simulink model "Filter"  (R2021a)
settings: Solver=VariableStepAuto  StartTime=0.0  StopTime=(len-1)*dt  FixedStep=0..005  RelTol=1e-3
values from neighbouring files (symbols this model uses):
  taos = 0.005    [Identify.m]    (also in Identify_time.m; Identify_wc.m)
  Wf = 10    [Identify.m]    (also in Identify_time.m; Identify_wc.m = Wf_list(i))
  zeta = 0.9    [Identify.m]    (also in Identify_time.m; Identify_wc.m)
settings Model: Creator=1  LastModifiedBy=1

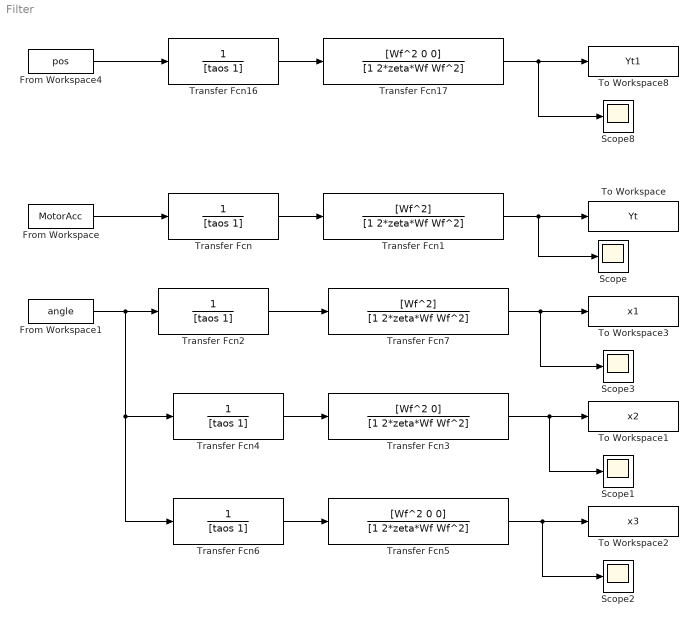
== system Filter ==
  From Workspace : FromWorkspace  VariableName=MotorAcc  OutDataTypeStr=double
  From Workspace1 : FromWorkspace  VariableName=angle  OutDataTypeStr=double
  From Workspace4 : FromWorkspace  VariableName=pos  OutDataTypeStr=double
  Scope{,1..3,8} (5 alike) : Scope
  To Workspace : ToWorkspace  VariableName=Yt  SampleTime=0.005
  To Workspace1 : ToWorkspace  VariableName=x2  SampleTime=0.005
  To Workspace2 : ToWorkspace  VariableName=x3  SampleTime=0.005
  To Workspace3 : ToWorkspace  VariableName=x1  SampleTime=0.005
  To Workspace8 : ToWorkspace  VariableName=Yt1  SampleTime=0.005
  Transfer Fcn{,2,4,6,16} (5 alike) : TransferFcn  Denominator=[taos 1]
  Transfer Fcn1 : TransferFcn  Numerator=[Wf^2]  Denominator=[1 2*zeta*Wf Wf^2]
  Transfer Fcn17 : TransferFcn  Numerator=[Wf^2 0 0]  Denominator=[1 2*zeta*Wf Wf^2]
  Transfer Fcn3 : TransferFcn  Numerator=[Wf^2 0]  Denominator=[1 2*zeta*Wf Wf^2]
  Transfer Fcn5 : TransferFcn  Numerator=[Wf^2 0 0]  Denominator=[1 2*zeta*Wf Wf^2]
  Transfer Fcn7 : TransferFcn  Numerator=[Wf^2]  Denominator=[1 2*zeta*Wf Wf^2]
  wires:
  From Workspace/1 -> Transfer Fcn/1
  Transfer Fcn7/1 -> Scope3/1, To Workspace3/1
  Transfer Fcn2/1 -> Transfer Fcn7/1
  From Workspace1/1 -> Transfer Fcn2/1, Transfer Fcn6/1, Transfer Fcn4/1
  Transfer Fcn/1 -> Transfer Fcn1/1
  Transfer Fcn1/1 -> Scope/1, To Workspace/1
  Transfer Fcn3/1 -> Scope1/1, To Workspace1/1
  Transfer Fcn4/1 -> Transfer Fcn3/1
  Transfer Fcn6/1 -> Transfer Fcn5/1
  Transfer Fcn5/1 -> Scope2/1, To Workspace2/1
  Transfer Fcn17/1 -> Scope8/1, To Workspace8/1
  Transfer Fcn16/1 -> Transfer Fcn17/1
  From Workspace4/1 -> Transfer Fcn16/1
